simulink model "Model_silnika"  (R2024a)
settings: Solver=VariableStepAuto  StartTime=0.0  StopTime=50  RelTol=1e-3
libraries: fuzblock x1, SignalEditorBlockLib x1
settings Model: SimulationMode=rapid-accelerator  Creator=kkucm  LastModifiedBy=krzysiek89
settings RTWCC: GPUComputeCapability=3.5

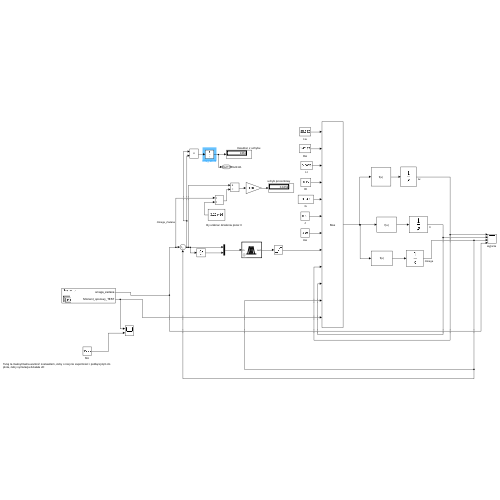
[thumbnail: Simulink's stored preview of the top-level diagram]
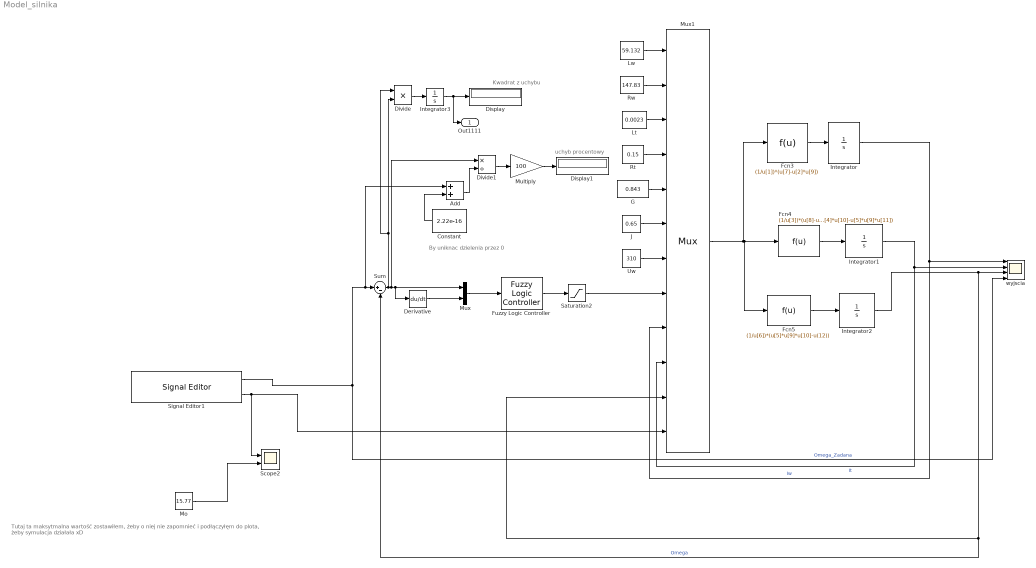
== system Model_silnika ==
  note: Tutaj ta maksytmalna wartość zostawiłem, żeby o niej nie zapomnieć i podłączyłęm do plota, żeby symulacja działała xD
  note: uchyb procentowy
  note: Kwadrat z uchybu
  note: By uniknac dzielenia przez 0
  Add : Sum
  Constant : Constant  Value=2.22e-16
  Derivative : Derivative
  Display : Display
  Display1 : Display
  Divide : Product  Inputs=**
  Divide1 : Product  Inputs=*/
  Fcn3 : Fcn  Expr=(1/u[1])*(u[7]-u[2]*u[9])
  Fcn4 : Fcn  Expr=(1/u[3])*(u[8]-u[4]*u[10]-u[5]*u[9]*u[11])
  Fcn5 : Fcn  Expr=(1/u[6])*(u[5]*u[9]*u[10]-u(12))
  Fuzzy Logic Controller : fuzblock/Fuzzy Logic  Controller  FIS='FuzzyC.fis'  OutputSampleNumber=101  DataType=double  FuzzifiedInputs=off  RuleFiringStrengths=off  RuleOutputs=off  AggregatedOutputs=off  SimulateUsing=Interpreted execution  OutOfRangeInputValueMessage=none  NoRuleFiredMessage=none  EmptyOutputFuzzySetMessage=none
  G : Constant  Value=0.843  VectorParams1D=off
  Integrator : Integrator
  Integrator1 : Integrator
  Integrator2 : Integrator
  Integrator3 : Integrator  LowerSaturationLimit=1e-5
  J : Constant  Value=0.65
  Lt : Constant  Value=0.0023
  Lw : Constant  Value=59.132
  Mo : Constant  Value=15.77
  Multiply : Gain  Gain=100
  Mux : Mux  Inputs=2
  Mux1 : Mux  Inputs=12
  Rt : Constant  Value=0.15
  Rw : Constant  Value=147.83
  Saturation2 : Saturate  UpperLimit=528  LowerLimit=0
  Scope2 : Scope  NumInputPorts=2
  Signal Editor1 : SignalEditorBlockLib/Signal Editor  FileName=omega_zadana.mat  ActiveScenario=Scenario  ActiveSignal=omaga_zadana  IsBus=off  OutputBusObjectStr=Bus: BusObject  SampleTime=0  ZeroCross=off  OutputAfterFinalValue=Setting to zero  Unit=inherit  PreserveSignalName=on  ApplySigPropsToAllScenarios=on  ApplySigPropsToAllSignals=off
  Sum : Sum  Inputs=|+-
  Uw : Constant  Value=310
  "wyjscia " : Scope  NumInputPorts=4
  Out1111 : Outport  SignalName=Out1111
  wires:
  Integrator/1 -> Mux1/9, "wyjscia "/1  "Iw"
  Uw/1 -> Mux1/7
  Mux1/1 -> Fcn3/1, Fcn5/1, Fcn4/1
  Integrator2/1 -> Mux1/11, Sum/2, "wyjscia "/3  "Omega"
  G/1 -> Mux1/5
  Integrator1/1 -> Mux1/10, "wyjscia "/2  "It"
  Lw/1 -> Mux1/1
  Lt/1 -> Mux1/3
  Rt/1 -> Mux1/4
  Saturation2/1 -> Mux1/8
  Fuzzy Logic Controller/1 -> Saturation2/1
  Rw/1 -> Mux1/2
  J/1 -> Mux1/6
  Fcn3/1 -> Integrator/1
  Fcn4/1 -> Integrator1/1
  Fcn5/1 -> Integrator2/1
  Derivative/1 -> Mux/2
  Mux/1 -> Fuzzy Logic Controller/1
  Mo/1 -> Scope2/2
  Signal Editor1/1 -> "wyjscia "/4, Add/1, Sum/1  "Omega_Zadana"
  Divide/1 -> Integrator3/1
  Divide1/1 -> Multiply/1
  Sum/1 -> Divide/1, Divide/2, Divide1/1, Derivative/1, Mux/1
  Add/1 -> Divide1/2
  Integrator3/1 -> Out1111/1, Display/1
  Constant/1 -> Add/2
  Multiply/1 -> Display1/1
  Signal Editor1/2 -> Mux1/12, Scope2/1
